simulink model "v22_receive"  (R2022a)
settings: Solver=FixedStepAuto  StartTime=0.0  StopTime=inf  FixedStep=0.1  RelTol=1e-3
model workspace (MAT data in the model file):
  Ki = 0.0002
  Kp = 0.05
  fc = 1200
  frameSymbols = 60
  fs = 9600
  refMagnitude = 2.99535
  rrcCoefficients = [0.00166950465783 0.00161541487245 0.00136077286171 0.000921868848776 0.000337964268746 -0.000331804375381 -0.00101405242267 -0.00162882202094 -0.00209855676539 -0.00235742969687 -0.00235997448449 -0.00208797727745 ... (129 elements, 1x129)]
  sps = 16
  squelch = 0.001
settings Model: Creator=luoch  LastModifiedBy=luoch
settings OptimizationCC: DefaultParameterBehavior=Inlined  EnhancedBackFolding=on  PassReuseOutputArgsAs=Individual arguments  ZeroExternalMemoryAtStartup=off  ZeroInternalMemoryAtStartup=off  OptimizeBlockOrder=speed  DifferentSizesBufferReuse=on  OptimizationCustomize=off  EfficientTunableParamExpr=on
settings DebuggingCC: ParameterTunabilityLossMsg=error
settings HardwareCC: ProdBitPerLong=64  ProdLargestAtomicInteger=LongLong  ProdLargestAtomicFloat=Double  ProdLongLongMode=on  ProdHWDeviceType=ARM Compatible->ARM Cortex-A (64-bit)
settings ModelReferenceCC: EnableRefExpFcnMdlSchedulingChecks=off
settings SFSimCC: MATLABDynamicMemAlloc=off
settings RTWCC: SystemTargetFile=ert.tlc  GenCodeOnly=on  TemplateMakefile=ert_default_tmf  GPUComputeCapability=5.0
settings CodeAppCC: ForceParamTrailComments=on  IgnoreCustomStorageClasses=off  OperatorAnnotations=on  SimulinkDataObjDesc=on  SFDataObjDesc=on  InsertBlockDesc=on
settings ERTTargetCC: TargetLangStandard=C99 (ISO)  InlinedParameterPlacement=NonHierarchical  RootIOFormat=Part of model data structure  ERTCustomFileTemplate=example_file_process.tlc
settings ConfigComp: CovBoundaryAbsTol=1.0e-5

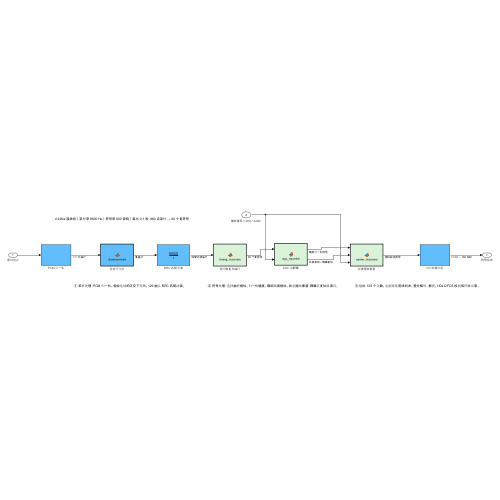
[thumbnail: Simulink's stored preview of the top-level diagram]
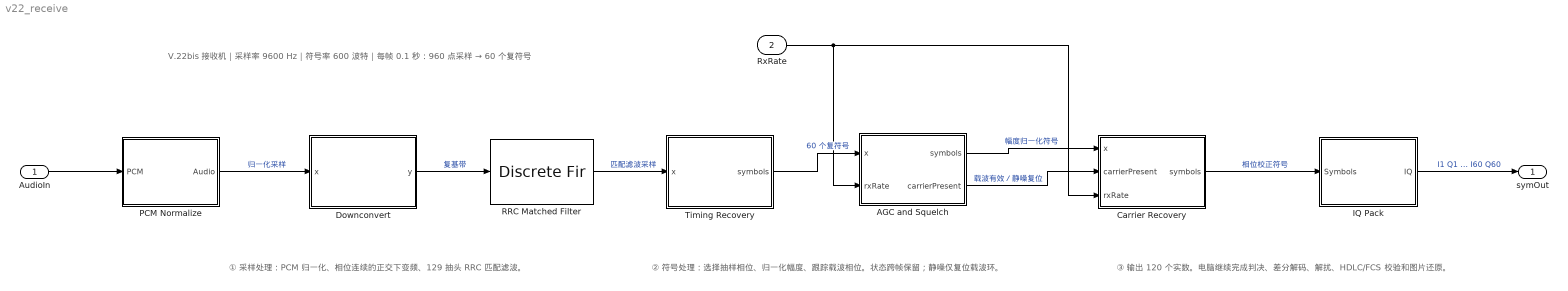
== system v22_receive ==
  note: V.22bis 接收机｜采样率 9600 Hz｜符号率 600 波特｜每帧 0.1 秒：960 点采样 → 60 个复符号
  note: ① 采样处理：PCM 归一化、相位连续的正交下变频、129 抽头 RRC 匹配滤波。
  note: ② 符号处理：选择抽样相位、归一化幅度、跟踪载波相位。状态跨帧保留；静噪仅复位载波环。
  note: ③ 输出 120 个实数。电脑继续完成判决、差分解码、解扰、HDLC/FCS 校验和图片还原。
  AudioIn : Inport  OutDataTypeStr=int16  PortDimensions=960  SampleTime=0.1
      settings: AttributesFormatString=音频输入
  RxRate : Inport  Port=2  OutDataTypeStr=uint16  PortDimensions=1  SampleTime=0.1
      settings: AttributesFormatString=接收速率（1200／2400）
  AGC and Squelch : MATLAB Function  Description=|  TreatAsAtomicUnit=on
      | 源文件: model/agc_squelch.m
      | 修改后运行 build_model 重新嵌入模型。
      settings: AttributesFormatString=AGC 与静噪
  Carrier Recovery : MATLAB Function  Description=|  TreatAsAtomicUnit=on
      | 源文件: model/carrier_recovery.m
      | 修改后运行 build_model 重新嵌入模型。
      settings: AttributesFormatString=载波相位恢复
  Downconvert : MATLAB Function  Description=|  TreatAsAtomicUnit=on
      | 源文件: model/downconvert.m
      | 修改后运行 build_model 重新嵌入模型。
      settings: AttributesFormatString=正交下变频
  IQ Pack : Subsystem
      settings: AttributesFormatString=I/Q 交替打包
  PCM Normalize : Subsystem
      settings: AttributesFormatString=PCM 归一化
  RRC Matched Filter : DiscreteFir  Coefficients=rrcCoefficients  InputProcessing=Columns as channels (frame based)
      settings: AttributesFormatString=RRC 匹配滤波
  Timing Recovery : MATLAB Function  Description=|  TreatAsAtomicUnit=on
      | 源文件: model/timing_recovery.m
      | 修改后运行 build_model 重新嵌入模型。
      settings: AttributesFormatString=定时恢复与抽样
  symOut : Outport
      settings: AttributesFormatString=符号输出
  wires:
  AudioIn/1 -> PCM Normalize/1(PCM)
  PCM Normalize/1(Audio) -> Downconvert/1(x)  "归一化采样"
  Downconvert/1(y) -> RRC Matched Filter/1  "复基带"
  RRC Matched Filter/1 -> Timing Recovery/1(x)  "匹配滤波采样"
  Timing Recovery/1(symbols) -> AGC and Squelch/1(x)  "60 个复符号"
  AGC and Squelch/1(symbols) -> Carrier Recovery/1(x)  "幅度归一化符号"
  Carrier Recovery/1(symbols) -> IQ Pack/1(Symbols)  "相位校正符号"
  IQ Pack/1(IQ) -> symOut/1  "I1 Q1 … I60 Q60"
  AGC and Squelch/2(carrierPresent) -> Carrier Recovery/2(carrierPresent)  "载波有效／静噪复位"
  RxRate/1 -> AGC and Squelch/2(rxRate), Carrier Recovery/3(rxRate)

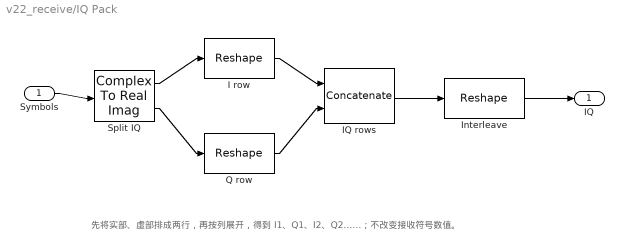
== system v22_receive/IQ Pack ==
  note: 先将实部、虚部排成两行，再按列展开，得到 I1、Q1、I2、Q2……；不改变接收符号数值。
  Symbols : Inport
      settings: AttributesFormatString=复符号
  I row : Reshape  OutputDimensionality=Customize  OutputDimensions=[1 60]
      settings: AttributesFormatString=实部行向量
  IQ rows : Concatenate  Mode=Multidimensional array
      settings: AttributesFormatString=上下拼成两行
  Interleave : Reshape
      settings: AttributesFormatString=按列展开
  Q row : Reshape  OutputDimensionality=Customize  OutputDimensions=[1 60]
      settings: AttributesFormatString=虚部行向量
  Split IQ : ComplexToRealImag
      settings: AttributesFormatString=分离实部与虚部
  IQ : Outport
      settings: AttributesFormatString=交替 I/Q
  wires:
  Symbols/1 -> Split IQ/1
  Split IQ/1 -> I row/1
  Split IQ/2 -> Q row/1
  I row/1 -> IQ rows/1
  Q row/1 -> IQ rows/2
  IQ rows/1 -> Interleave/1
  Interleave/1 -> IQ/1

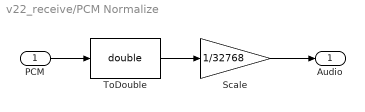
== system v22_receive/PCM Normalize ==
  PCM : Inport
      settings: AttributesFormatString=整数音频
  Scale : Gain  Gain=1/32768
      settings: AttributesFormatString=除以 32768
  ToDouble : DataTypeConversion  OutDataTypeStr=double  SaturateOnIntegerOverflow=off  RndMeth=Floor
      settings: AttributesFormatString=转为双精度
  Audio : Outport
      settings: AttributesFormatString=归一化音频
  wires:
  PCM/1 -> ToDouble/1
  ToDouble/1 -> Scale/1
  Scale/1 -> Audio/1

== matlab function v22_receive/Timing Recovery ==
  data: x input; symbols output; sps parameter; frameSymbols parameter
function symbols = timing_recovery(x, sps, frameSymbols)
%#codegen
% 16 个候选抽样相位：按帧平滑幅度和，再选最大者抽取 60 个符号。
% 状态跨帧保留；静噪时也继续更新，保持旧接收机的定时行为。
persistent energy
if isempty(energy),energy=zeros(sps,1);end
SPS=int32(sps);NS=int32(frameSymbols);
for p=1:SPS
    total=0;
    for k=1:NS
        total=total+abs(x(int32(p)+(k-1)*SPS));
    end
    energy(p)=0.9*energy(p)+0.1*total;
end
phase=int32(1);best=energy(1);
for p=2:SPS
    if energy(p)>best,best=energy(p);phase=int32(p);end
end
symbols=complex(zeros(frameSymbols,1));
for k=1:NS,symbols(k)=x(phase+(k-1)*SPS);end
end

== matlab function v22_receive/Downconvert ==
  data: x input; y output; fc parameter; fs parameter
function y = downconvert(x, fc, fs)
%#codegen
% 连续相位下变频：输入实数采样帧，输出同长度复基带。
persistent phase
if isempty(phase), phase=0; end
step=2*pi*fc/fs;
y=complex(zeros(size(x)));
for k=1:numel(x)
    y(k)=x(k)*complex(cos(-phase),sin(-phase))*2;
    phase=phase+step;
    if phase>2*pi,phase=phase-2*pi;end
end
end

== matlab function v22_receive/AGC and Squelch ==
  data: x input; symbols output; rxRate input; carrierPresent output; refMagnitude parameter; squelch parameter
function [symbols, carrierPresent] = agc_squelch(x, rxRate, refMagnitude, squelch)
%#codegen
% 按当前 60 符号帧归一化；门限以下输出零，并通知载波环复位。
meanMagnitude=0;
for k=1:numel(x),meanMagnitude=meanMagnitude+abs(x(k));end
meanMagnitude=meanMagnitude/double(numel(x));
carrierPresent=meanMagnitude>squelch;
% QPSK 为单位圆；16-QAM 保留原有平均幅度。
if rxRate==1200,refMagnitude=1;end
if carrierPresent,gain=refMagnitude/meanMagnitude;else,gain=0;end
symbols=complex(zeros(size(x)));
for k=1:numel(x),symbols(k)=x(k)*gain;end
end

== matlab function v22_receive/Carrier Recovery ==
  data: x input; symbols output; carrierPresent input; rxRate input; Kp parameter; Ki parameter
function symbols = carrier_recovery(x, carrierPresent, rxRate, Kp, Ki)
%#codegen
% 二阶判决引导载波环。输出校正后的实收符号，不输出理想判决点。
% 每个符号更新环路；跨帧保存相位/积分，在静噪、重新捕获或切档时复位。
persistent phase integral wasActive previousRate
if isempty(phase),phase=0;integral=0;wasActive=false;previousRate=rxRate;end
if ~carrierPresent || ~wasActive || rxRate~=previousRate,phase=0;integral=0;end
wasActive=carrierPresent;previousRate=rxRate;
reference=[1+1i,3+1i,1+3i,3+3i];
symbols=complex(zeros(size(x)));
for k=1:numel(x)
    z=x(k)*complex(cos(-phase),sin(-phase));
    re=real(z);im=imag(z);
    if re>=0 && im>=0,quadrant=0;
    elseif re<0 && im>=0,quadrant=1;
    elseif re<0 && im<0,quadrant=2;
    else,quadrant=3;
    end
    a=-pi/2*double(quadrant);
    firstQuadrant=z*complex(cos(a),sin(a));
    if rxRate==1200
        % QPSK 每个象限只有对角线一个点，避免锁到 16-QAM 的非对角点。
        firstDecision=complex(1/sqrt(2),1/sqrt(2));
    else
        bestIndex=1;bestDistance=inf;
        for q=1:4
            distance=abs(firstQuadrant-reference(q));
            if distance<bestDistance,bestDistance=distance;bestIndex=q;end
        end
        firstDecision=reference(bestIndex);
    end
    decision=firstDecision*complex(cos(-a),sin(-a));
    error=angle(z*conj(decision));
    integral=integral+Ki*error;
    phase=phase+Kp*error+integral;
    symbols(k)=z;
end
end
